simulink model "theorycontrolHW2Q2Simulink"  (R2024a)
settings: Solver=VariableStepAuto  StartTime=0.0  StopTime=10.0  RelTol=1e-3

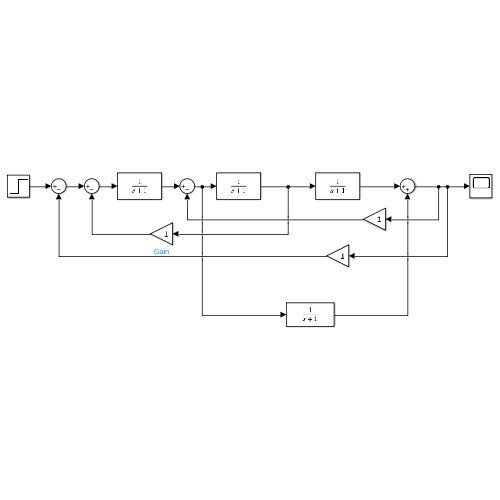
[thumbnail: Simulink's stored preview of the top-level diagram]
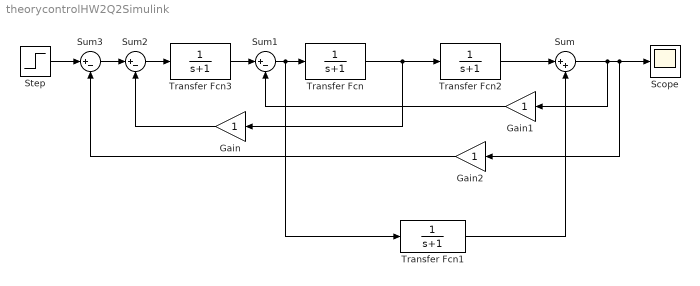
== system theorycontrolHW2Q2Simulink ==
  Gain : Gain
  Gain1 : Gain
  Gain2 : Gain
  Scope : Scope
  Step : Step  SampleTime=0
  Sum : Sum  Inputs=|++
  Sum1 : Sum  Inputs=|+-
  Sum2 : Sum  Inputs=|+-
  Sum3 : Sum  Inputs=|+-
  Transfer Fcn{,1..3} (4 alike) : TransferFcn  Denominator=[1 1]
  wires:
  Transfer Fcn3/1 -> Sum1/1
  Transfer Fcn/1 -> Gain/1, Transfer Fcn2/1
  Transfer Fcn2/1 -> Sum/1
  Sum2/1 -> Transfer Fcn3/1
  Sum3/1 -> Sum2/1
  Step/1 -> Sum3/1
  Gain1/1 -> Sum1/2
  Sum/1 -> Scope/1, Gain2/1, Gain1/1
  Gain2/1 -> Sum3/2
  Gain/1 -> Sum2/2
  Sum1/1 -> Transfer Fcn1/1, Transfer Fcn/1
  Transfer Fcn1/1 -> Sum/2
